simulink model "SimulinkforArduinoTest"  (R2013b)
settings: Solver=ode45  StartTime=0.0  StopTime=500  RelTol=1e-3
libraries: arduino_io_lib x2
settings Model: Creator=gyurse  LastModifiedBy=gyurse

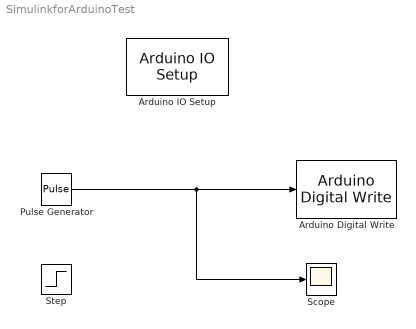
== system SimulinkforArduinoTest ==
  Arduino Digital Write : arduino_io_lib/Arduino Digital Write  arduinoVar=Existing workspace arduino variable #1  arduinoPin=13  T=0.2
  Arduino IO Setup : arduino_io_lib/Arduino IO Setup  Priority=3  arduinoVar=Existing workspace arduino variable #1  workspaceVarName=a  comPort=COM3
  Pulse Generator : DiscretePulseGenerator  PulseType=Time based  Period=100  PulseWidth=50
  Scope : Scope
  Step : Step  SampleTime=0
  wires:
  Pulse Generator/1 -> Scope/1, Arduino Digital Write/1
